simulink model "UGV_collison_avoidance_LiDAR_example1"  (R2024b)
settings: Solver=FixedStepAuto  StartTime=0.0  StopTime=inf  RelTol=1e-3  EnableMultiTasking=on
values from neighbouring files (symbols this model uses):
  RC_max = 2000    [Init_collision_avoidance_UGV.m]
  RC_min = 1000    [Init_collision_avoidance_UGV.m]
libraries: px4Peripheralslib x1, px4Sensorslib x1, px4uORBlib x1
settings Model: ExtModeTrigDuration=10  Creator=ADMIN  LastModifiedBy=User
settings SolverCC: PositivePriorityOrder=on
settings OptimizationCC: EnhancedBackFolding=on  PassReuseOutputArgsAs=Individual arguments  ZeroExternalMemoryAtStartup=off  ZeroInternalMemoryAtStartup=off  MaxStackSize=64  OptimizeBlockOrder=speed  DifferentSizesBufferReuse=on  OptimizationCustomize=off  EfficientTunableParamExpr=on
settings DebuggingCC: ParameterTunabilityLossMsg=error
settings HardwareCC: ProdBitPerPointer=32  ProdBitPerSizeT=32  ProdBitPerPtrDiffT=32  ProdLargestAtomicInteger=Long  ProdLargestAtomicFloat=Double  ProdWordSize=32  ProdLongLongMode=on  ProdHWDeviceType=ARM Compatible->ARM Cortex
settings SFSimCC: MATLABDynamicMemAlloc=off  SimTargetLang=C++
settings RTWCC: Description=Embedded Coder  SystemTargetFile=ert.tlc  HardwareBoard=PX4 Pixhawk 6x  TLCOptions="-aInlineSetEventsForThisBaseRateFcn=TLC_FALSE -aSuppressMultiTaskScheduler=TLC_FALSE  -aRateBasedStepFcn=0"  TemplateMakefile=ert_default_tmf  Toolchain=GNU Tools for PX4 Autopilots  TargetLang=C++  GPUComputeCapability=3.5
settings CodeAppCC: ForceParamTrailComments=on  IgnoreCustomStorageClasses=off  OperatorAnnotations=on  SimulinkDataObjDesc=on  SFDataObjDesc=on  InsertBlockDesc=on
settings ERTTargetCC: ExtModeTransport=3  ExtModeStaticAlloc=on  ExtModeStaticAllocSize=1024  ExtModeMexFile=ext_xcp  ExtModeIntrfLevel=Level2 - Open  InlinedParameterPlacement=Hierarchical  DynamicArrayContainerType=coder::array

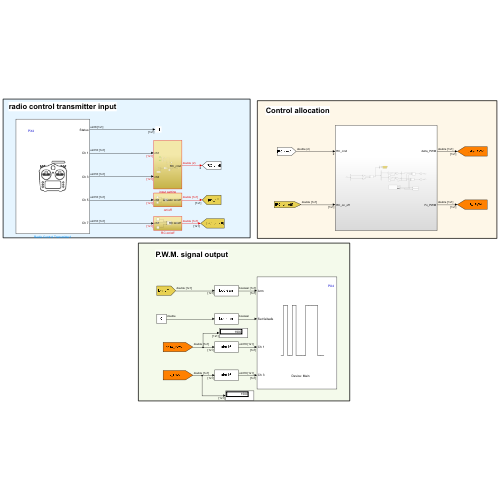
[thumbnail: Simulink's stored preview of the top-level diagram]
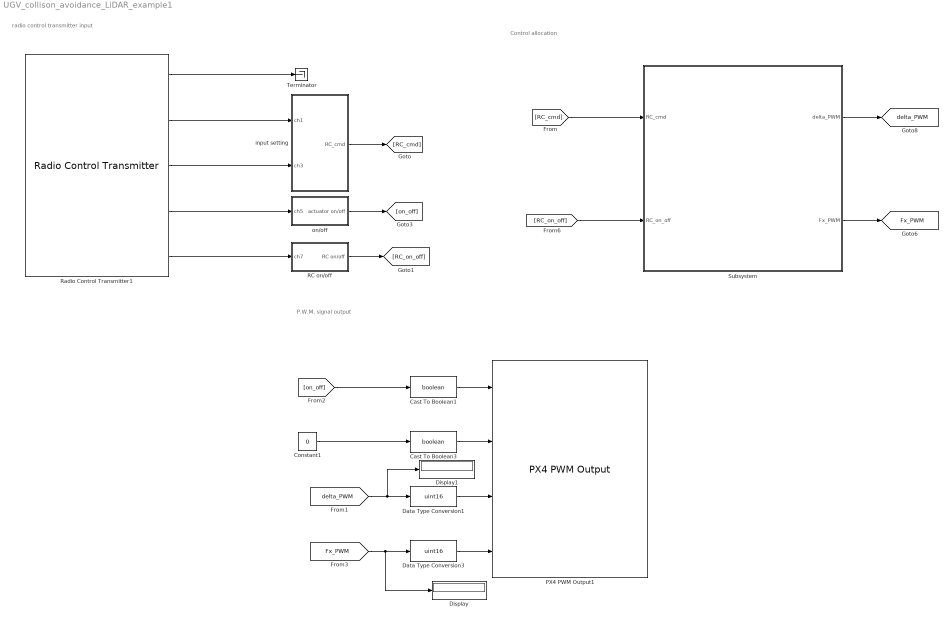
== system UGV_collison_avoidance_LiDAR_example1 ==
  note: P.W.M. signal output
  note: Control allocation
  note: radio control transmitter input
  Cast To Boolean1 : DataTypeConversion  OutDataTypeStr=boolean  SaturateOnIntegerOverflow=off  RndMeth=Floor
  Cast To Boolean3 : DataTypeConversion  OutDataTypeStr=boolean  SaturateOnIntegerOverflow=off  RndMeth=Floor
  Constant1 : Constant  Value=0
  Data Type Conversion1 : DataTypeConversion  OutDataTypeStr=uint16  SaturateOnIntegerOverflow=off  RndMeth=Floor
  Data Type Conversion3 : DataTypeConversion  OutDataTypeStr=uint16  SaturateOnIntegerOverflow=off  RndMeth=Floor
  Display : Display
  Display1 : Display
  PX4 PWM Output1 : px4Peripheralslib/PX4 PWM Output  pwmDevice=Main  pwmChannel1_=on  pwmChannel2_=off  pwmChannel3_=on  pwmChannel4_=off  pwmChannel5_=off  pwmChannel6_=off  pwmChannel7_=off  pwmChannel8_=off
      settings: SourceProductName=PX4 Peripheral Blocks
  RC on/off : Subsystem
  Radio Control Transmitter1 : px4Sensorslib/Radio Control Transmitter  channel1=on  channel2=off  channel3=on  channel4=off  channel5=on  channel6=off  channel7=on  channel8=off  channel_count=off  rssi=off  rc_input_source=off  timestamp_last_signal=off  time_stamp=off  sampleTime=1/250  BlockingMode=off  BlockTimeout=5
  Subsystem : Subsystem
  Terminator : Terminator
  input setting : Subsystem
  on/off : Subsystem
  tag scope: Fx_PWM=global, delta_PWM=global
  wires:
  [on_off] -> Cast To Boolean1/1
  Constant1/1 -> Cast To Boolean3/1
  Cast To Boolean1/1 -> PX4 PWM Output1/1
  Cast To Boolean3/1 -> PX4 PWM Output1/2
  Data Type Conversion1/1 -> PX4 PWM Output1/3
  Data Type Conversion3/1 -> PX4 PWM Output1/4
  input setting/1(RC_cmd) -> [RC_cmd]
  Radio Control Transmitter1/2 -> input setting/1(ch1)
  Radio Control Transmitter1/5 -> RC on/off/1(ch7)
  Subsystem/1(delta_PWM) -> [delta_PWM]
  Radio Control Transmitter1/4 -> on/off/1(ch5)
  on/off/1(actuator on/off) -> [on_off]
  Subsystem/2(Fx_PWM) -> [Fx_PWM]
  [RC_cmd] -> Subsystem/1(RC_cmd)
  RC on/off/1(RC on/off) -> [RC_on_off]
  Radio Control Transmitter1/1 -> Terminator/1
  Radio Control Transmitter1/3 -> input setting/2(ch3)
  [delta_PWM] -> Display1/1, Data Type Conversion1/1
  [Fx_PWM] -> Display/1, Data Type Conversion3/1
  [RC_on_off] -> Subsystem/2(RC_on_off)

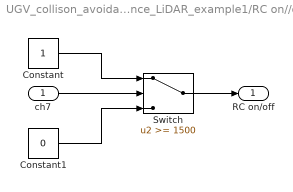
== system UGV_collison_avoidance_LiDAR_example1/RC on//off ==
  ch7 : Inport
  Constant : Constant
  Constant1 : Constant  Value=0
  Switch : Switch  Threshold=1500  SaturateOnIntegerOverflow=off  InputSameDT=off
  RC on/off : Outport
  wires:
  Switch/1 -> RC on/off/1
  ch7/1 -> Switch/2
  Constant/1 -> Switch/1
  Constant1/1 -> Switch/3

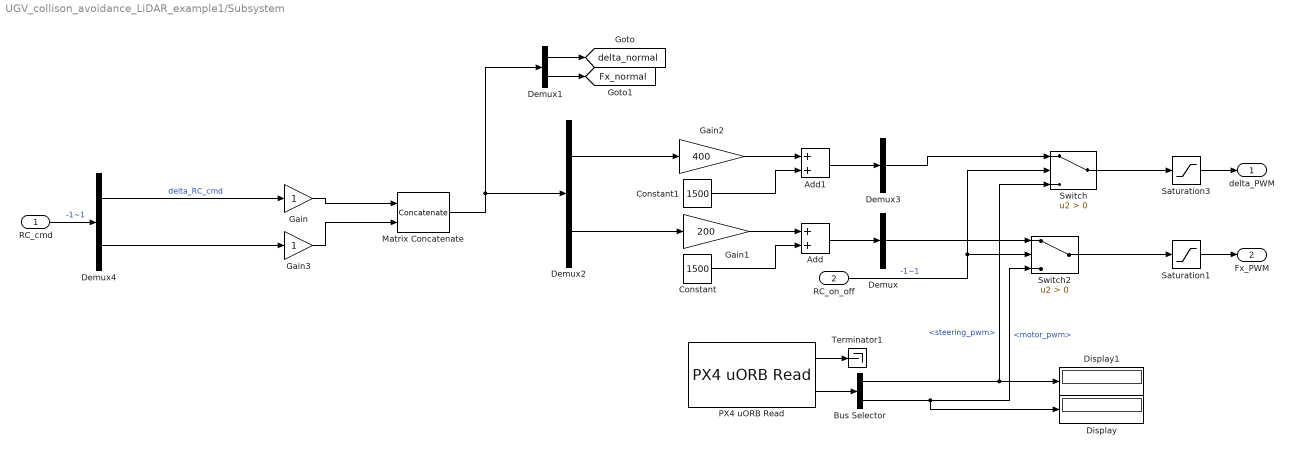
== system UGV_collison_avoidance_LiDAR_example1/Subsystem ==
  RC_cmd : Inport
  RC_on_off : Inport  Port=2
  Add : Sum
  Add1 : Sum
  Bus Selector : BusSelector  OutputSignals=steering_pwm,motor_pwm
  Constant : Constant  Value=1500
  Constant1 : Constant  Value=1500
  Demux : Demux  Outputs=1
  Demux1 : Demux  Outputs=2
  Demux2 : Demux  Outputs=2
  Demux3 : Demux  Outputs=1
  Demux4 : Demux  Outputs=2
  Display : Display
  Display1 : Display
  Gain : Gain
  Gain1 : Gain  Gain=200
  Gain2 : Gain  Gain=400
  Gain3 : Gain
  Matrix Concatenate : Concatenate  Mode=Multidimensional array
  PX4 uORB Read : px4uORBlib/PX4 uORB Read  uORBTopic=ActuatorCommand  selectInstance=ActuatorCommand  SampleTime=-1  BlockingMode=off  BlockTimeout=1e-3
  Saturation1 : Saturate  UpperLimit=1700  LowerLimit=1300
  Saturation3 : Saturate  UpperLimit=1900  LowerLimit=1100
  Switch : Switch  Criteria=u2 > Threshold  SaturateOnIntegerOverflow=off  InputSameDT=off
  Switch2 : Switch  Criteria=u2 > Threshold  SaturateOnIntegerOverflow=off  InputSameDT=off
  Terminator1 : Terminator
  delta_PWM : Outport
  Fx_PWM : Outport  Port=2
  tag scope: Fx_normal=global, delta_normal=global
  wires:
  Demux4/2 -> Gain3/1
  Demux1/1 -> [delta_normal]
  Demux1/2 -> [Fx_normal]
  Matrix Concatenate/1 -> Demux1/1, Demux2/1
  Gain/1 -> Matrix Concatenate/1
  Gain3/1 -> Matrix Concatenate/2
  Add/1 -> Demux/1
  Gain1/1 -> Add/1
  Constant/1 -> Add/2
  Constant1/1 -> Add1/2
  Add1/1 -> Demux3/1
  Gain2/1 -> Add1/1
  Demux2/1 -> Gain2/1
  Demux2/2 -> Gain1/1
  RC_cmd/1 -> Demux4/1  "-1~1"
  PX4 uORB Read/1 -> Terminator1/1
  PX4 uORB Read/2 -> Bus Selector/1
  Bus Selector/1 -> Switch/3, Display1/1  "<steering_pwm>"
  Bus Selector/2 -> Display/1, Switch2/3  "<motor_pwm>"
  RC_on_off/1 -> Switch2/2, Switch/2  "-1~1"
  Demux3/1 -> Switch/1
  Demux/1 -> Switch2/1
  Switch/1 -> Saturation3/1
  Switch2/1 -> Saturation1/1
  Demux4/1 -> Gain/1  "delta_RC_cmd"
  Saturation3/1 -> delta_PWM/1
  Saturation1/1 -> Fx_PWM/1

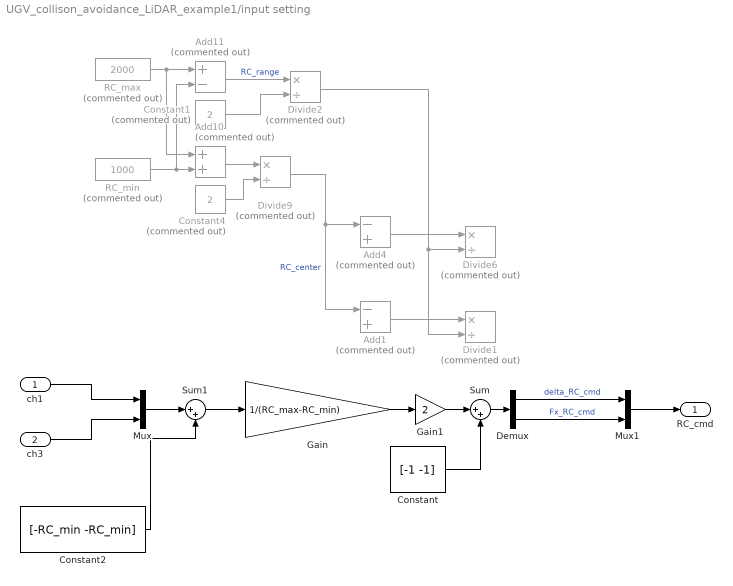
== system UGV_collison_avoidance_LiDAR_example1/input setting ==
  ch1 : Inport
  ch3 : Inport  Port=2
  Add1 : Sum  Commented=on  Inputs=-+  OutDataTypeStr=single
  Add10 : Sum  Commented=on
  Add11 : Sum  Commented=on  Inputs=+-
  Add4 : Sum  Commented=on  Inputs=-+  OutDataTypeStr=single
  Constant : Constant  Value=[-1 -1]
  Constant1 : Constant  Commented=on  Value=2  OutDataTypeStr=single
  Constant2 : Constant  Value=[-RC_min -RC_min]
  Constant4 : Constant  Commented=on  Value=2  OutDataTypeStr=single
  Demux : Demux  Outputs=2
  Divide{1..2,6,9} (4 alike) : Product  Commented=on  Inputs=*/
  Gain : Gain  Gain=1/(RC_max-RC_min)
  Gain1 : Gain  Gain=2
  Mux : Mux  Inputs=2
  Mux1 : Mux  Inputs=2
  RC_max : Constant  Commented=on  Value=2000  OutDataTypeStr=int16
  RC_min : Constant  Commented=on  Value=1000  OutDataTypeStr=int16
  Sum : Sum  Inputs=|++
  Sum1 : Sum  Inputs=|++
  RC_cmd : Outport
  wires:
  Constant4/1 -> Divide9/2
  Add10/1 -> Divide9/1
  Constant1/1 -> Divide2/2
  Add11/1 -> Divide2/1  "RC_range"
  RC_max/1 -> Add10/1, Add11/1
  RC_min/1 -> Add11/2, Add10/2
  ch1/1 -> Mux/1
  Divide9/1 -> Add1/1, Add4/1  "RC_center"
  Add4/1 -> Divide6/1
  Divide2/1 -> Divide1/2, Divide6/2
  ch3/1 -> Mux/2
  Add1/1 -> Divide1/1
  Gain/1 -> Gain1/1
  Mux/1 -> Sum1/1
  Gain1/1 -> Sum/1
  Sum1/1 -> Gain/1
  Sum/1 -> Demux/1
  Demux/1 -> Mux1/1  "delta_RC_cmd"
  Demux/2 -> Mux1/2  "Fx_RC_cmd"
  Constant/1 -> Sum/2
  Constant2/1 -> Sum1/2
  Mux1/1 -> RC_cmd/1

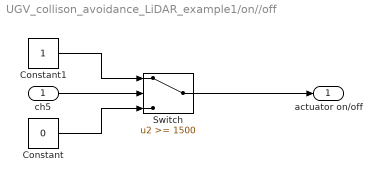
== system UGV_collison_avoidance_LiDAR_example1/on//off ==
  ch5 : Inport
  Constant : Constant  Value=0
  Constant1 : Constant
  Switch : Switch  Threshold=1500  SaturateOnIntegerOverflow=off  InputSameDT=off
  actuator on/off : Outport
  wires:
  Constant1/1 -> Switch/1
  Constant/1 -> Switch/3
  ch5/1 -> Switch/2
  Switch/1 -> actuator on/off/1
